simulink model "CtrlStrct_CAN_Variant"  (R2018a)
settings: Solver=VariableStepAuto  StartTime=0.0  StopTime=10.0  FixedStep=sampletime  RelTol=1e-3  EnableMultiTasking=on
PreLoadFcn:
  | CtrlStrct_SmplCAN_BusInfo
undefined symbols (not defined in the file or in its folder): canChannel
libraries: canmsglib x106, canlib x35, simulink x1
(part 2 of 8)

== system CtrlStrct_CAN_Variant/CAN_Variant/Simple_CAN_TW/HEV_Ctrl ==
  note: HEV control
  note: HEV control
  note: CAN receive and transmit
  Bus Creator1 : BusCreator  Inputs=13
  Bus Selector3 : BusSelector  OutputSignals=BatteryCtrl_PwtrCAN_Tx.BatCtrl_SOC,TransmCtrl_PwtrCAN_Tx.TmCtrl_Clutch_position,TransmCtrl_PwtrCAN_Tx.TmCtrl_Gear_position,Gateway_PwtrCAN_Tx.BrkCtrl_Vehicle_speed,Gateway_PwtrCAN_Tx.BrkCtrl_Regen_brake_torque_request,MotorCtrl_PwtrCAN_Tx.MtrCtrl_Motor_torque_actual,MotorCtrl_PwtrCAN_Tx.MtrCtrl_Motor_torque_available,MotorCtrl_PwtrCAN_Tx.MtrCtrl_Motor_regen_torque_available,EngineCtrl_PwtrCAN_Tx.EngCtrl_Engine_speed,EngineCtrl_PwtrCAN_Tx.EngCtrl_Engine_torque_actual,Gateway_PwtrCAN_Tx.VMCtrl_PropTorqStatus,Gateway_PwtrCAN_Tx.VMCtrl_PropTorqCmnd,Gateway_PwtrCAN_Tx.NAVI_Home_around_status
  Rate Transition1 : RateTransition  Deterministic=off
      settings: AttributesFormatString=<Deterministic=%<Deterministic>>
  Rate Transition2 : RateTransition  Deterministic=off
      settings: AttributesFormatString=<Deterministic=%<Deterministic>>
  Two-Way Connection : TwoWayConnection
  HevCtrl_PwtrCAN : PMIOPort  Side=Left
      settings: AttributesFormatString=<Side=%<Side>>
  tag scope: HEV_Ctrl_PwtrCAN_Rx=scoped
  wires:
  [HEV_Ctrl_PwtrCAN_Tx] -> Rate Transition2/1
  Bus Creator1/1 -> Rate Transition1/1
  Two-Way Connection/1 -> Bus Selector3/1
  Rate Transition1/1 -> [HEV_Ctrl_PwtrCAN_Rx]  "HEV_Ctrl_PwtrCAN_Rx"
  Rate Transition2/1 -> Two-Way Connection/1  "HEV_Ctrl_PwtrCAN_Tx"
  Bus Selector3/1 -> Bus Creator1/1  "<BatCtrl_SOC>"
  Bus Selector3/2 -> Bus Creator1/2  "<TmCtrl_Clutch_position>"
  Bus Selector3/3 -> Bus Creator1/3  "<TmCtrl_Gear_position>"
  Bus Selector3/4 -> Bus Creator1/4  "<BrkCtrl_Vehicle_speed>"
  Bus Selector3/5 -> Bus Creator1/5  "<BrkCtrl_Regen_brake_torque_request>"
  Bus Selector3/6 -> Bus Creator1/6  "<MtrCtrl_Motor_torque_actual>"
  Bus Selector3/7 -> Bus Creator1/7  "<MtrCtrl_Motor_torque_available>"
  Bus Selector3/8 -> Bus Creator1/8  "<MtrCtrl_Motor_regen_torque_available>"
  Bus Selector3/9 -> Bus Creator1/9  "<EngCtrl_Engine_speed>"
  Bus Selector3/10 -> Bus Creator1/10  "<EngCtrl_Engine_torque_actual>"
  Bus Selector3/11 -> Bus Creator1/11  "<VMCtrl_PropTorqStatus>"
  Bus Selector3/12 -> Bus Creator1/12  "<VMCtrl_PropTorqCmnd>"
  Bus Selector3/13 -> Bus Creator1/13  "<NAVI_Home_around_status>"
  connections:
  HevCtrl_PwtrCAN/RConn1 -- Two-Way Connection/RConn1

== system CtrlStrct_CAN_Variant/CAN_Variant/Simple_CAN_TW/HVAC_Ctrl ==
  note: HVAC control
  note: CAN receive and transmit
  note: HVAC Control
  Bus Creator : BusCreator  Inputs=3
  Bus Selector : BusSelector  OutputSignals=Gateway_VehCAN_Tx.EngCtrl_Engine_speed,Gateway_VehCAN_Tx.HEVCtrl_IdleStop_preparation_request,Gateway_VehCAN_Tx.HEVCtrl_IdleStop_status
  Rate Transition1 : RateTransition  Deterministic=off
      settings: AttributesFormatString=<Deterministic=%<Deterministic>>
  Rate Transition2 : RateTransition  Deterministic=off
      settings: AttributesFormatString=<Deterministic=%<Deterministic>>
  Two-Way Connection : TwoWayConnection
  HVAC_Ctrl_VehCAN : PMIOPort  Side=Right
      settings: AttributesFormatString=<Side=%<Side>>
  tag scope: HVAC_Ctrl_VehCAN_Rx=scoped
  wires:
  [HVAC_Ctrl_VehCAN_Tx] -> Rate Transition2/1
  Bus Creator/1 -> Rate Transition1/1
  Two-Way Connection/1 -> Bus Selector/1
  Rate Transition1/1 -> [HVAC_Ctrl_VehCAN_Rx]  "HVAC_Ctrl_VehCAN_Rx"
  Rate Transition2/1 -> Two-Way Connection/1  "HVAC_Ctrl_VehCAN_Tx"
  Bus Selector/3 -> Bus Creator/3  "<HEVCtrl_IdleStop_status>"
  Bus Selector/2 -> Bus Creator/2  "<HEVCtrl_IdleStop_preparation_request>"
  Bus Selector/1 -> Bus Creator/1  "<EngCtrl_Engine_speed>"
  connections:
  HVAC_Ctrl_VehCAN/RConn1 -- Two-Way Connection/RConn1

== system CtrlStrct_CAN_Variant/CAN_Variant/Simple_CAN_TW/InfoCAN ==
  note: Infotainment CAN
  Bus Creator : BusCreator  Inputs=3
  InfoCAN_Memory : Memory
  Two-Way Connection : TwoWayConnection
  Two-Way Connection1 : TwoWayConnection
  Two-Way Connection2 : TwoWayConnection
  NAVI_InfoCAN : PMIOPort  Side=Left
      settings: AttributesFormatString=<Side=%<Side>>
  Radar_InfoCAN : PMIOPort  Port=2  Side=Left
      settings: AttributesFormatString=<Side=%<Side>>
  Gateway_InfoCAN : PMIOPort  Port=3  Side=Right
      settings: AttributesFormatString=<Side=%<Side>>
  wires:
  Bus Creator/1 -> InfoCAN_Memory/1  "InfoCAN"
  InfoCAN_Memory/1 -> Two-Way Connection1/1, Two-Way Connection/1, Two-Way Connection2/1  "InfoCAN"
  Two-Way Connection/1 -> Bus Creator/2
  Two-Way Connection1/1 -> Bus Creator/3
  Two-Way Connection2/1 -> Bus Creator/1
  connections:
  Two-Way Connection/RConn1 -- NAVI_InfoCAN/RConn1
  Two-Way Connection1/RConn1 -- Radar_InfoCAN/RConn1
  Two-Way Connection2/RConn1 -- Gateway_InfoCAN/RConn1

== system CtrlStrct_CAN_Variant/CAN_Variant/Simple_CAN_TW/Motor_Ctrl ==
  note: Motor control
  note: Motor Control
  note: CAN receive and transmit
  Bus Creator7 : BusCreator  Inputs=3
  Bus Selector2 : BusSelector  OutputSignals=TransmCtrl_PwtrCAN_Tx.TmCtrl_Clutch_position,HEV_Ctrl_PwtrCAN_Tx.HEVCtrl_Motor_torque_request,EngineCtrl_PwtrCAN_Tx.EngCtrl_Engine_speed
  Rate Transition1 : RateTransition  Deterministic=off
      settings: AttributesFormatString=<Deterministic=%<Deterministic>>
  Rate Transition2 : RateTransition  Deterministic=off
      settings: AttributesFormatString=<Deterministic=%<Deterministic>>
  Two-Way Connection : TwoWayConnection
  MtrCtrl_PwtrCAN : PMIOPort  Side=Left
      settings: AttributesFormatString=<Side=%<Side>>
  tag scope: MotorCtrl_PwtrCAN_Rx=scoped
  wires:
  [MotorCtrl_PwtrCAN_Tx] -> Rate Transition2/1
  Rate Transition1/1 -> [MotorCtrl_PwtrCAN_Rx]  "MotorCtrl_PwtrCAN_Rx"
  Bus Selector2/3 -> Bus Creator7/3  "<EngCtrl_Engine_speed>"
  Bus Creator7/1 -> Rate Transition1/1
  Bus Selector2/1 -> Bus Creator7/1  "<TmCtrl_Clutch_position>"
  Bus Selector2/2 -> Bus Creator7/2  "<HEVCtrl_Motor_torque_request>"
  Two-Way Connection/1 -> Bus Selector2/1
  Rate Transition2/1 -> Two-Way Connection/1  "MotorCtrl_PwtrCAN_Tx"
  connections:
  MtrCtrl_PwtrCAN/RConn1 -- Two-Way Connection/RConn1

== system CtrlStrct_CAN_Variant/CAN_Variant/Simple_CAN_TW/NAVI ==
  note: Navigation
  note: Navigation
  note: CAN receive and transmit
  Bus Creator : BusCreator  Inputs=1
  Bus Selector1 : BusSelector  OutputSignals=Gateway_InfoCAN_Tx.BrkCtrl_Vehicle_speed
  Rate Transition1 : RateTransition  Deterministic=off
      settings: AttributesFormatString=<Deterministic=%<Deterministic>>
  Rate Transition2 : RateTransition  Deterministic=off
      settings: AttributesFormatString=<Deterministic=%<Deterministic>>
  Two-Way Connection : TwoWayConnection
  NAVI_InfoCAN : PMIOPort  Side=Right
      settings: AttributesFormatString=<Side=%<Side>>
  tag scope: NAVI_InfoCAN_Rx=scoped
  wires:
  [NAVI_InfoCAN_Tx] -> Rate Transition2/1
  Two-Way Connection/1 -> Bus Selector1/1
  Bus Selector1/1 -> Bus Creator/1  "<BrkCtrl_Vehicle_speed>"
  Bus Creator/1 -> Rate Transition1/1
  Rate Transition1/1 -> [NAVI_InfoCAN_Rx]  "NAVI_InfoCAN_Rx"
  Rate Transition2/1 -> Two-Way Connection/1  "NAVI_InfoCAN_Tx"
  connections:
  NAVI_InfoCAN/RConn1 -- Two-Way Connection/RConn1

== system CtrlStrct_CAN_Variant/CAN_Variant/Simple_CAN_TW/PwtrCAN ==
  note: Powertrain CAN
  Bus Creator3 : BusCreator  Inputs=6
  PwtrCAN_Memory : Memory
  Two-Way Connection{,1..5} (6 alike) : TwoWayConnection
  Gateway_PwtrCAN : PMIOPort  Side=Left
      settings: AttributesFormatString=<Side=%<Side>>
  HevCtrl_PwtrCAN : PMIOPort  Port=2  Side=Right
      settings: AttributesFormatString=<Side=%<Side>>
  EngCtrl_PwtrCAN : PMIOPort  Port=3  Side=Right
      settings: AttributesFormatString=<Side=%<Side>>
  TrsmCtrl_PwtrCAN : PMIOPort  Port=4  Side=Right
      settings: AttributesFormatString=<Side=%<Side>>
  MtrCtrl_PwtrCAN : PMIOPort  Port=5  Side=Right
      settings: AttributesFormatString=<Side=%<Side>>
  BatCtrl_PwtrCAN : PMIOPort  Port=6  Side=Right
      settings: AttributesFormatString=<Side=%<Side>>
  wires:
  Bus Creator3/1 -> PwtrCAN_Memory/1  "PwtrCAN"
  PwtrCAN_Memory/1 -> Two-Way Connection5/1, Two-Way Connection4/1, Two-Way Connection3/1, Two-Way Connection2/1, Two-Way Connection1/1, Two-Way Connection/1  "PwtrCAN"
  Two-Way Connection1/1 -> Bus Creator3/2
  Two-Way Connection/1 -> Bus Creator3/1
  Two-Way Connection2/1 -> Bus Creator3/3
  Two-Way Connection5/1 -> Bus Creator3/6
  Two-Way Connection4/1 -> Bus Creator3/5
  Two-Way Connection3/1 -> Bus Creator3/4
  connections:
  Two-Way Connection/RConn1 -- Gateway_PwtrCAN/RConn1
  HevCtrl_PwtrCAN/RConn1 -- Two-Way Connection1/RConn1
  EngCtrl_PwtrCAN/RConn1 -- Two-Way Connection2/RConn1
  Two-Way Connection3/RConn1 -- TrsmCtrl_PwtrCAN/RConn1
  MtrCtrl_PwtrCAN/RConn1 -- Two-Way Connection4/RConn1
  BatCtrl_PwtrCAN/RConn1 -- Two-Way Connection5/RConn1

== system CtrlStrct_CAN_Variant/CAN_Variant/Simple_CAN_TW/Radar ==
  note: Radar detection
  note: CAN receive and transmit
  note: Radar Detection
  Bus Creator : BusCreator  Inputs=1
  Bus Selector1 : BusSelector  OutputSignals=Gateway_InfoCAN_Tx.BrkCtrl_Vehicle_speed
  Rate Transition1 : RateTransition  Deterministic=off
      settings: AttributesFormatString=<Deterministic=%<Deterministic>>
  Rate Transition2 : RateTransition  Deterministic=off
      settings: AttributesFormatString=<Deterministic=%<Deterministic>>
  Two-Way Connection : TwoWayConnection
  Radar_InfoCAN : PMIOPort  Side=Right
      settings: AttributesFormatString=<Side=%<Side>>
  tag scope: Radar_InfoCAN_Rx=scoped
  wires:
  [Radar_InfoCAN_Tx] -> Rate Transition2/1
  Bus Selector1/1 -> Bus Creator/1  "<BrkCtrl_Vehicle_speed>"
  Bus Creator/1 -> Rate Transition1/1
  Two-Way Connection/1 -> Bus Selector1/1
  Rate Transition1/1 -> [Radar_InfoCAN_Rx]  "Radar_InfoCAN_Rx"
  Rate Transition2/1 -> Two-Way Connection/1  "Radar_InfoCAN_Tx"
  connections:
  Radar_InfoCAN/RConn1 -- Two-Way Connection/RConn1

== system CtrlStrct_CAN_Variant/CAN_Variant/Simple_CAN_TW/Steer_Ctrl ==
  note: Steering control
  note: CAN receive and transmit
  note: Steering Control
  Bus Creator : BusCreator  Inputs=1
  Bus Selector1 : BusSelector  OutputSignals=BrakeCtrl_VehCAN_Tx.BrkCtrl_Vehicle_speed
  Rate Transition1 : RateTransition  Deterministic=off
      settings: AttributesFormatString=<Deterministic=%<Deterministic>>
  Rate Transition2 : RateTransition  Deterministic=off
      settings: AttributesFormatString=<Deterministic=%<Deterministic>>
  Two-Way Connection : TwoWayConnection
  StrCtrl_VehCAN : PMIOPort  Side=Right
      settings: AttributesFormatString=<Side=%<Side>>
  tag scope: SteerCtrl_VehCAN_Rx=scoped
  wires:
  [SteerCtrl_VehCAN_Tx] -> Rate Transition2/1
  Bus Selector1/1 -> Bus Creator/1  "<BrkCtrl_Vehicle_speed>"
  Bus Creator/1 -> Rate Transition1/1
  Two-Way Connection/1 -> Bus Selector1/1
  Rate Transition1/1 -> [SteerCtrl_VehCAN_Rx]  "SteerCtrl_VehCAN_Rx"
  Rate Transition2/1 -> Two-Way Connection/1  "SteerCtrl_VehCAN_Tx"
  connections:
  StrCtrl_VehCAN/RConn1 -- Two-Way Connection/RConn1

== system CtrlStrct_CAN_Variant/CAN_Variant/Simple_CAN_TW/Transms_Ctrl ==
  note: Transmission control
  note: Transmission Control
  note: CAN receive and transmit
  Bus Creator6 : BusCreator  Inputs=2
  Bus Selector1 : BusSelector  OutputSignals=Gateway_PwtrCAN_Tx.BrkCtrl_Vehicle_speed,EngineCtrl_PwtrCAN_Tx.EngCtrl_Engine_speed
  Rate Transition1 : RateTransition  Deterministic=off
      settings: AttributesFormatString=<Deterministic=%<Deterministic>>
  Rate Transition2 : RateTransition  Deterministic=off
      settings: AttributesFormatString=<Deterministic=%<Deterministic>>
  Two-Way Connection : TwoWayConnection
  TrsmCtrl_PwtrCAN : PMIOPort  Side=Left
      settings: AttributesFormatString=<Side=%<Side>>
  tag scope: TransmCtrl_PwtrCAN_Rx=scoped
  wires:
  [TransmCtrl_PwtrCAN_Tx] -> Rate Transition2/1
  Rate Transition2/1 -> Two-Way Connection/1  "TransmCtrl_PwtrCAN_Tx"
  Bus Selector1/1 -> Bus Creator6/1  "<BrkCtrl_Vehicle_speed>"
  Bus Creator6/1 -> Rate Transition1/1
  Bus Selector1/2 -> Bus Creator6/2  "<EngCtrl_Engine_speed>"
  Two-Way Connection/1 -> Bus Selector1/1
  Rate Transition1/1 -> [TransmCtrl_PwtrCAN_Rx]  "TransmCtrl_PwtrCAN_Rx"
  connections:
  TrsmCtrl_PwtrCAN/RConn1 -- Two-Way Connection/RConn1

== system CtrlStrct_CAN_Variant/CAN_Variant/Simple_CAN_TW/VM_Ctrl ==
  note: Vehicle motion control
  note: Vehicle Motion Control
  note: CAN receive and transmit
  Bus Creator : BusCreator  Inputs=1
  Bus Selector1 : BusSelector  OutputSignals=BrakeCtrl_VehCAN_Tx.BrkCtrl_Vehicle_speed
  Rate Transition1 : RateTransition  Deterministic=off
      settings: AttributesFormatString=<Deterministic=%<Deterministic>>
  Rate Transition2 : RateTransition  Deterministic=off
      settings: AttributesFormatString=<Deterministic=%<Deterministic>>
  Two-Way Connection : TwoWayConnection
  VM_Ctrl_VehCAN : PMIOPort  Side=Right
      settings: AttributesFormatString=<Side=%<Side>>
  tag scope: VM_Ctrl_VehCAN_Rx=scoped
  wires:
  [VM_Ctrl_VehCAN_Tx] -> Rate Transition2/1
  Bus Selector1/1 -> Bus Creator/1  "<BrkCtrl_Vehicle_speed>"
  Bus Creator/1 -> Rate Transition1/1
  Two-Way Connection/1 -> Bus Selector1/1
  Rate Transition1/1 -> [VM_Ctrl_VehCAN_Rx]  "VM_Ctrl_VehCAN_Rx"
  Rate Transition2/1 -> Two-Way Connection/1  "VM_Ctrl_VehCAN_Tx"
  connections:
  VM_Ctrl_VehCAN/RConn1 -- Two-Way Connection/RConn1

== system CtrlStrct_CAN_Variant/CAN_Variant/Simple_CAN_TW/VehCAN ==
  note: Vehicle CAN
  Bus Creator1 : BusCreator  Inputs=6
  Two-Way Connection{,1..5} (6 alike) : TwoWayConnection
  VehCAN_Memory : Memory
  Gateway_VehCAN : PMIOPort  Side=Right
      settings: AttributesFormatString=<Side=%<Side>>
  VM_Ctrl_VehCAN : PMIOPort  Port=2  Side=Left
      settings: AttributesFormatString=<Side=%<Side>>
  BrkCtrl_VehCAN : PMIOPort  Port=3  Side=Left
      settings: AttributesFormatString=<Side=%<Side>>
  StrCtrl_VehCAN : PMIOPort  Port=4  Side=Left
      settings: AttributesFormatString=<Side=%<Side>>
  HVAC_Ctrl_VehCAN : PMIOPort  Port=5  Side=Left
      settings: AttributesFormatString=<Side=%<Side>>
  BdyCtrl_VehCAN : PMIOPort  Port=6  Side=Left
      settings: AttributesFormatString=<Side=%<Side>>
  wires:
  Bus Creator1/1 -> VehCAN_Memory/1  "VehCAN"
  Two-Way Connection3/1 -> Bus Creator1/4
  Two-Way Connection1/1 -> Bus Creator1/2
  Two-Way Connection5/1 -> Bus Creator1/6
  VehCAN_Memory/1 -> Two-Way Connection/1, Two-Way Connection3/1, Two-Way Connection2/1, Two-Way Connection1/1, Two-Way Connection4/1, Two-Way Connection5/1  "VehCAN"
  Two-Way Connection2/1 -> Bus Creator1/3
  Two-Way Connection/1 -> Bus Creator1/1
  Two-Way Connection4/1 -> Bus Creator1/5
  connections:
  Gateway_VehCAN/RConn1 -- Two-Way Connection/RConn1
  Two-Way Connection1/RConn1 -- VM_Ctrl_VehCAN/RConn1
  Two-Way Connection2/RConn1 -- BrkCtrl_VehCAN/RConn1
  Two-Way Connection3/RConn1 -- StrCtrl_VehCAN/RConn1
  Two-Way Connection4/RConn1 -- HVAC_Ctrl_VehCAN/RConn1
  BdyCtrl_VehCAN/RConn1 -- Two-Way Connection5/RConn1

== system CtrlStrct_CAN_Variant/CAN_Variant/VNT_Level1_CAN_TW/Battery_Ctrl ==
  note: Battery control
  note: CAN receive and transmit
  note: Battery Control
  BatteryCtrl_PwtrCAN Tx : Subsystem
  BatteryCtrl_PwtrCAN_Rx : Subsystem
  Two-Way Connection : TwoWayConnection
  BatCtrl_PwtrCAN : PMIOPort  Side=Left
      settings: AttributesFormatString=<Side=%<Side>>
  tag scope: BatteryCtrl_PwtrCAN_Rx=scoped
  wires:
  [BatteryCtrl_PwtrCAN_Tx] -> BatteryCtrl_PwtrCAN Tx/1(BatteryCtrl_PwtrCAN_Tx_Apli)
  BatteryCtrl_PwtrCAN_Rx/1(BatteryCtrl_PwtrCAN_Rx) -> [BatteryCtrl_PwtrCAN_Rx]
  Two-Way Connection/1 -> BatteryCtrl_PwtrCAN_Rx/1(PwtrCAN)
  BatteryCtrl_PwtrCAN Tx/1(BatteryCtrl_PwtrCAN_Tx) -> Two-Way Connection/1
  connections:
  BatCtrl_PwtrCAN/RConn1 -- Two-Way Connection/RConn1

== system CtrlStrct_CAN_Variant/CAN_Variant/VNT_Level1_CAN_TW/Body_Ctrl ==
  note: Body control
  note: Body Control
  note: CAN receive and transmit
  BodyCtrl_VehCAN Tx : Subsystem
  BodyCtrl_VehCAN_Rx : Subsystem
  Two-Way Connection : TwoWayConnection
  BdyCtrl_VehCAN : PMIOPort  Side=Right
      settings: AttributesFormatString=<Side=%<Side>>
  tag scope: BodyCtrl_VehCAN_Rx=scoped
  wires:
  [BodyCtrl_VehCAN_Tx] -> BodyCtrl_VehCAN Tx/1(BodyCtrl_VehCAN_Tx_Apli)
  BodyCtrl_VehCAN_Rx/1(BodyCtrl_VehCAN_Rx) -> [BodyCtrl_VehCAN_Rx]
  Two-Way Connection/1 -> BodyCtrl_VehCAN_Rx/1(VehCAN)
  BodyCtrl_VehCAN Tx/1(BodyCtrl_VehCAN_Tx) -> Two-Way Connection/1
  connections:
  BdyCtrl_VehCAN/RConn1 -- Two-Way Connection/RConn1

== system CtrlStrct_CAN_Variant/CAN_Variant/VNT_Level1_CAN_TW/Brake_Ctrl ==
  note: Brake control
  note: Brake Control
  note: CAN receive and transmit
  BrakeCtrl_VehCAN Tx : Subsystem
  BrakeCtrl_VehCAN_Rx : Subsystem
  Two-Way Connection : TwoWayConnection
  BrkCtrl_VehCAN : PMIOPort  Side=Right
      settings: AttributesFormatString=<Side=%<Side>>
  tag scope: BrakeCtrl_VehCAN_Rx=scoped
  wires:
  [BrakeCtrl_VehCAN_Tx] -> BrakeCtrl_VehCAN Tx/1(BrakeCtrl_VehCAN_Tx_Apli)
  BrakeCtrl_VehCAN_Rx/1(BrakeCtrl_VehCAN_Rx) -> [BrakeCtrl_VehCAN_Rx]
  Two-Way Connection/1 -> BrakeCtrl_VehCAN_Rx/1(VehCAN)
  BrakeCtrl_VehCAN Tx/1(BrakeCtrl_VehCAN_Tx) -> Two-Way Connection/1
  connections:
  BrkCtrl_VehCAN/RConn1 -- Two-Way Connection/RConn1

== system CtrlStrct_CAN_Variant/CAN_Variant/VNT_Level1_CAN_TW/Engine_Ctrl ==
  note: Engine control
  note: Engine Control
  note: CAN receive and transmit
  EngineCtrl_PwtrCAN Tx : Subsystem
  EngineCtrl_PwtrCAN_Rx : Subsystem
  Two-Way Connection : TwoWayConnection
  EngCtrl_PwtrCAN : PMIOPort  Side=Left
      settings: AttributesFormatString=<Side=%<Side>>
  tag scope: EngineCtrl_PwtrCAN_Rx=scoped
  wires:
  [EngineCtrl_PwtrCAN_Tx] -> EngineCtrl_PwtrCAN Tx/1(EngineCtrl_PwtrCAN_Tx_Apli)
  EngineCtrl_PwtrCAN_Rx/1(EngineCtrl_PwtrCAN_Rx) -> [EngineCtrl_PwtrCAN_Rx]
  Two-Way Connection/1 -> EngineCtrl_PwtrCAN_Rx/1(PwtrCAN)
  EngineCtrl_PwtrCAN Tx/1(EngineCtrl_PwtrCAN_Tx) -> Two-Way Connection/1
  connections:
  EngCtrl_PwtrCAN/RConn1 -- Two-Way Connection/RConn1

== system CtrlStrct_CAN_Variant/CAN_Variant/VNT_Level1_CAN_TW/Gateway ==
  note: Gateway
  Gateway InfoCAN : Subsystem
  Gateway PwtrCAN : Subsystem
  Gateway VehCAN : Subsystem
  Info Hub : Subsystem
  Two-Way Connection : TwoWayConnection
  Two-Way Connection1 : TwoWayConnection
  Two-Way Connection2 : TwoWayConnection
  Gateway_InfoCAN : PMIOPort  Side=Left
      settings: AttributesFormatString=<Side=%<Side>>
  Gateway_VehCAN : PMIOPort  Port=2  Side=Left
      settings: AttributesFormatString=<Side=%<Side>>
  Gateway_PwtrCAN : PMIOPort  Port=3  Side=Right
      settings: AttributesFormatString=<Side=%<Side>>
  wires:
  Two-Way Connection1/1 -> Gateway PwtrCAN/2(VehCAN), Gateway InfoCAN/1(VehCAN), Info Hub/2(VehCAN)
  Two-Way Connection2/1 -> Gateway VehCAN/2(PwtrCAN), Info Hub/3(PwtrCAN)
  Two-Way Connection/1 -> Gateway VehCAN/1(InfoCAN), Gateway PwtrCAN/1(InfoCAN), Info Hub/1(InfoCAN)
  Gateway InfoCAN/1(Gateway_InfoCAN) -> Two-Way Connection/1
  Gateway VehCAN/1(Gateway_VehCAN_Tx) -> Two-Way Connection1/1
  Gateway PwtrCAN/1(Gateway_PwtrCAN_Tx) -> Two-Way Connection2/1
  connections:
  Gateway_InfoCAN/RConn1 -- Two-Way Connection/RConn1
  Two-Way Connection1/RConn1 -- Gateway_VehCAN/RConn1
  Gateway_PwtrCAN/RConn1 -- Two-Way Connection2/RConn1

== system CtrlStrct_CAN_Variant/CAN_Variant/VNT_Level1_CAN_TW/HEV_Ctrl ==
  note: HEV control
  note: HEV control
  note: CAN receive and transmit
  HEV_Ctrl_PwtrCAN Tx : Subsystem
  HEV_Ctrl_PwtrCAN_Rx : Subsystem
  Two-Way Connection : TwoWayConnection
  HevCtrl_PwtrCAN : PMIOPort  Side=Left
      settings: AttributesFormatString=<Side=%<Side>>
  tag scope: HEV_Ctrl_PwtrCAN_Rx=scoped
  wires:
  [HEV_Ctrl_PwtrCAN_Tx] -> HEV_Ctrl_PwtrCAN Tx/1(HEV_Ctrl_PwtrCAN_Tx_Apli)
  Two-Way Connection/1 -> HEV_Ctrl_PwtrCAN_Rx/1(PwtrCAN)
  HEV_Ctrl_PwtrCAN_Rx/1(HEV_Ctrl_PwtrCAN_Rx) -> [HEV_Ctrl_PwtrCAN_Rx]
  HEV_Ctrl_PwtrCAN Tx/1(HEV_Ctrl_PwtrCAN_Tx) -> Two-Way Connection/1
  connections:
  HevCtrl_PwtrCAN/RConn1 -- Two-Way Connection/RConn1

== system CtrlStrct_CAN_Variant/CAN_Variant/VNT_Level1_CAN_TW/HVAC_Ctrl ==
  note: HVAC control
  note: CAN receive and transmit
  note: HVAC Control
  HVAC_Ctrl_VehCAN Tx : Subsystem
  HVAC_Ctrl_VehCAN_Rx : Subsystem
  Two-Way Connection : TwoWayConnection
  HVAC_Ctrl_VehCAN : PMIOPort  Side=Right
      settings: AttributesFormatString=<Side=%<Side>>
  tag scope: HVAC_Ctrl_VehCAN_Rx=scoped
  wires:
  [HVAC_Ctrl_VehCAN_Tx] -> HVAC_Ctrl_VehCAN Tx/1(HVAC_Ctrl_VehCAN_Tx_Apli)
  Two-Way Connection/1 -> HVAC_Ctrl_VehCAN_Rx/1(VehCAN)
  HVAC_Ctrl_VehCAN_Rx/1(HVAC_Ctrl_VehCAN_Rx) -> [HVAC_Ctrl_VehCAN_Rx]
  HVAC_Ctrl_VehCAN Tx/1(HVAC_Ctrl_VehCAN_Tx) -> Two-Way Connection/1
  connections:
  HVAC_Ctrl_VehCAN/RConn1 -- Two-Way Connection/RConn1

== system CtrlStrct_CAN_Variant/CAN_Variant/VNT_Level1_CAN_TW/InfoCAN ==
  note: Infotainment CAN
  Bus Creator : BusCreator  Inputs=3
  Bus Selector : BusSelector  OutputSignals=NAVI_InfoCAN_Tx_0CFFB01C
  Bus Selector1 : BusSelector  OutputSignals=Gateway_InfoCAN_Tx_0CFFC485
  Bus Selector2 : BusSelector  OutputSignals=Radar_InfoCAN_Tx_0CFF0080
  CAN_Memory : Memory
  Two-Way Connection : TwoWayConnection
  Two-Way Connection1 : TwoWayConnection
  Two-Way Connection2 : TwoWayConnection
  NAVI_InfoCAN : PMIOPort  Side=Left
      settings: AttributesFormatString=<Side=%<Side>>
  Radar_InfoCAN : PMIOPort  Port=2  Side=Left
      settings: AttributesFormatString=<Side=%<Side>>
  Gateway_InfoCAN : PMIOPort  Port=3  Side=Right
      settings: AttributesFormatString=<Side=%<Side>>
  wires:
  Bus Creator/1 -> CAN_Memory/1  "InfoCAN"
  CAN_Memory/1 -> Two-Way Connection2/1, Two-Way Connection1/1, Two-Way Connection/1  "InfoCAN"
  Two-Way Connection/1 -> Bus Selector/1
  Two-Way Connection1/1 -> Bus Selector2/1
  Two-Way Connection2/1 -> Bus Selector1/1
  Bus Selector1/1 -> Bus Creator/1  "<Gateway_InfoCAN_Tx_0CFFC485>"
  Bus Selector/1 -> Bus Creator/2  "<NAVI_InfoCAN_Tx_0CFFB01C>"
  Bus Selector2/1 -> Bus Creator/3  "<Radar_InfoCAN_Tx_0CFF0080>"
  connections:
  Two-Way Connection/RConn1 -- NAVI_InfoCAN/RConn1
  Two-Way Connection1/RConn1 -- Radar_InfoCAN/RConn1
  Two-Way Connection2/RConn1 -- Gateway_InfoCAN/RConn1

== system CtrlStrct_CAN_Variant/CAN_Variant/VNT_Level1_CAN_TW/Motor_Ctrl ==
  note: Motor control
  note: Motor Control
  note: CAN receive and transmit
  MotorCtrl_PwtrCAN Tx : Subsystem
  MotorCtrl_PwtrCAN_Rx : Subsystem
  Two-Way Connection : TwoWayConnection
  MtrCtrl_PwtrCAN : PMIOPort  Side=Left
      settings: AttributesFormatString=<Side=%<Side>>
  tag scope: MotorCtrl_PwtrCAN_Rx=scoped
  wires:
  [MotorCtrl_PwtrCAN_Tx] -> MotorCtrl_PwtrCAN Tx/1(IMotorCtrl_PwtrCAN_Tx_Apli)
  Two-Way Connection/1 -> MotorCtrl_PwtrCAN_Rx/1(PwtrCAN)
  MotorCtrl_PwtrCAN_Rx/1(MotorCtrl_PwtrCAN_Rx) -> [MotorCtrl_PwtrCAN_Rx]
  MotorCtrl_PwtrCAN Tx/1(MotorCtrl_PwtrCAN_Tx_0CFF5083) -> Two-Way Connection/1
  connections:
  MtrCtrl_PwtrCAN/RConn1 -- Two-Way Connection/RConn1

== system CtrlStrct_CAN_Variant/CAN_Variant/VNT_Level1_CAN_TW/NAVI ==
  note: Navigation
  note: Navigation
  note: CAN receive and transmit
  NAVI_InfoCAN_Rx : Subsystem
  NAVI_InfoCAN_Tx : Subsystem
  Two-Way Connection : TwoWayConnection
  NAVI_InfoCAN : PMIOPort  Side=Right
      settings: AttributesFormatString=<Side=%<Side>>
  tag scope: NAVI_InfoCAN_Rx=scoped
  wires:
  Two-Way Connection/1 -> NAVI_InfoCAN_Rx/1(InfoCAN)
  NAVI_InfoCAN_Rx/1(NAVI_InfoCAN_Rx) -> [NAVI_InfoCAN_Rx]
  [NAVI_InfoCAN_Tx] -> NAVI_InfoCAN_Tx/1(NAVI_InfoCAN_Tx_Apli)
  NAVI_InfoCAN_Tx/1(NAVI_InfoCAN_Tx) -> Two-Way Connection/1
  connections:
  NAVI_InfoCAN/RConn1 -- Two-Way Connection/RConn1

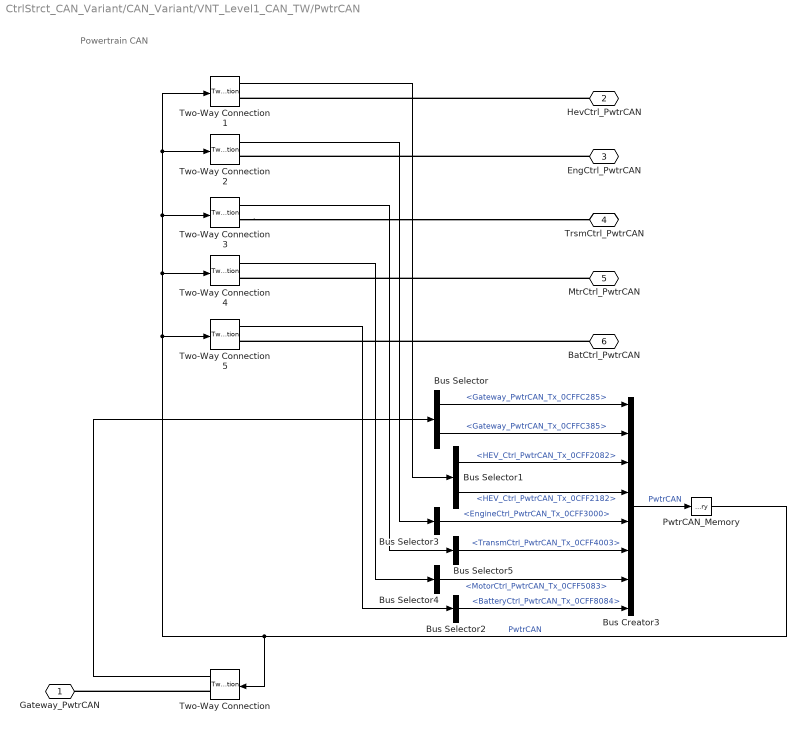
== system CtrlStrct_CAN_Variant/CAN_Variant/VNT_Level1_CAN_TW/PwtrCAN ==
  note: Powertrain CAN
  Bus Creator3 : BusCreator  Inputs=8
  Bus Selector : BusSelector  OutputSignals=Gateway_PwtrCAN_Tx_0CFFC285,Gateway_PwtrCAN_Tx_0CFFC385
  Bus Selector1 : BusSelector  OutputSignals=HEV_Ctrl_PwtrCAN_Tx_0CFF2082,HEV_Ctrl_PwtrCAN_Tx_0CFF2182
  Bus Selector2 : BusSelector  OutputSignals=BatteryCtrl_PwtrCAN_Tx_0CFF8084
  Bus Selector3 : BusSelector  OutputSignals=EngineCtrl_PwtrCAN_Tx_0CFF3000
  Bus Selector4 : BusSelector  OutputSignals=MotorCtrl_PwtrCAN_Tx_0CFF5083
  Bus Selector5 : BusSelector  OutputSignals=TransmCtrl_PwtrCAN_Tx_0CFF4003
  PwtrCAN_Memory : Memory
  Two-Way Connection{,1..5} (6 alike) : TwoWayConnection
  Gateway_PwtrCAN : PMIOPort  Side=Left
      settings: AttributesFormatString=<Side=%<Side>>
  HevCtrl_PwtrCAN : PMIOPort  Port=2  Side=Right
      settings: AttributesFormatString=<Side=%<Side>>
  EngCtrl_PwtrCAN : PMIOPort  Port=3  Side=Right
      settings: AttributesFormatString=<Side=%<Side>>
  TrsmCtrl_PwtrCAN : PMIOPort  Port=4  Side=Right
      settings: AttributesFormatString=<Side=%<Side>>
  MtrCtrl_PwtrCAN : PMIOPort  Port=5  Side=Right
      settings: AttributesFormatString=<Side=%<Side>>
  BatCtrl_PwtrCAN : PMIOPort  Port=6  Side=Right
      settings: AttributesFormatString=<Side=%<Side>>
  wires:
  Bus Creator3/1 -> PwtrCAN_Memory/1  "PwtrCAN"
  PwtrCAN_Memory/1 -> Two-Way Connection5/1, Two-Way Connection4/1, Two-Way Connection3/1, Two-Way Connection2/1, Two-Way Connection1/1, Two-Way Connection/1  "PwtrCAN"
  Two-Way Connection1/1 -> Bus Selector1/1
  Two-Way Connection/1 -> Bus Selector/1
  Two-Way Connection2/1 -> Bus Selector3/1
  Two-Way Connection5/1 -> Bus Selector2/1
  Two-Way Connection4/1 -> Bus Selector4/1
  Two-Way Connection3/1 -> Bus Selector5/1
  Bus Selector/1 -> Bus Creator3/1  "<Gateway_PwtrCAN_Tx_0CFFC285>"
  Bus Selector/2 -> Bus Creator3/2  "<Gateway_PwtrCAN_Tx_0CFFC385>"
  Bus Selector1/1 -> Bus Creator3/3  "<HEV_Ctrl_PwtrCAN_Tx_0CFF2082>"
  Bus Selector1/2 -> Bus Creator3/4  "<HEV_Ctrl_PwtrCAN_Tx_0CFF2182>"
  Bus Selector3/1 -> Bus Creator3/5  "<EngineCtrl_PwtrCAN_Tx_0CFF3000>"
  Bus Selector5/1 -> Bus Creator3/6  "<TransmCtrl_PwtrCAN_Tx_0CFF4003>"
  Bus Selector4/1 -> Bus Creator3/7  "<MotorCtrl_PwtrCAN_Tx_0CFF5083>"
  Bus Selector2/1 -> Bus Creator3/8  "<BatteryCtrl_PwtrCAN_Tx_0CFF8084>"
  connections:
  Two-Way Connection/RConn1 -- Gateway_PwtrCAN/RConn1
  HevCtrl_PwtrCAN/RConn1 -- Two-Way Connection1/RConn1
  EngCtrl_PwtrCAN/RConn1 -- Two-Way Connection2/RConn1
  Two-Way Connection3/RConn1 -- TrsmCtrl_PwtrCAN/RConn1
  MtrCtrl_PwtrCAN/RConn1 -- Two-Way Connection4/RConn1
  BatCtrl_PwtrCAN/RConn1 -- Two-Way Connection5/RConn1

== system CtrlStrct_CAN_Variant/CAN_Variant/VNT_Level1_CAN_TW/Radar ==
  note: Radar detection
  note: CAN receive and transmit
  note: Radar Detection
  Radar_InfoCAN_Rx : Subsystem
  Radar_InfoCAN_Tx : Subsystem
  Two-Way Connection : TwoWayConnection
  Radar_InfoCAN : PMIOPort  Side=Right
      settings: AttributesFormatString=<Side=%<Side>>
  tag scope: Radar_InfoCAN_Rx=scoped
  wires:
  Two-Way Connection/1 -> Radar_InfoCAN_Rx/1(InfoCAN)
  Radar_InfoCAN_Rx/1(Radar_InfoCAN_Rx) -> [Radar_InfoCAN_Rx]
  [Radar_InfoCAN_Tx] -> Radar_InfoCAN_Tx/1(Radar_InfoCAN_Tx_Apli)
  Radar_InfoCAN_Tx/1(Radar_InfoCAN_Tx) -> Two-Way Connection/1
  connections:
  Radar_InfoCAN/RConn1 -- Two-Way Connection/RConn1

== system CtrlStrct_CAN_Variant/CAN_Variant/VNT_Level1_CAN_TW/Steer_Ctrl ==
  note: Steering control
  note: CAN receive and transmit
  note: Steering Control
  SteerCtrl_VehCAN Tx : Subsystem
  SteerCtrl_VehCAN_Rx : Subsystem
  Two-Way Connection : TwoWayConnection
  StrCtrl_VehCAN : PMIOPort  Side=Right
      settings: AttributesFormatString=<Side=%<Side>>
  tag scope: SteerCtrl_VehCAN_Rx=scoped
  wires:
  [SteerCtrl_VehCAN_Tx] -> SteerCtrl_VehCAN Tx/1(SteerCtrl_VehCAN_Tx_Apli)
  Two-Way Connection/1 -> SteerCtrl_VehCAN_Rx/1(VehCAN)
  SteerCtrl_VehCAN_Rx/1(SteerCtrl_VehCAN_Rx) -> [SteerCtrl_VehCAN_Rx]
  SteerCtrl_VehCAN Tx/1(SteerCtrl_VehCAN_Tx) -> Two-Way Connection/1
  connections:
  StrCtrl_VehCAN/RConn1 -- Two-Way Connection/RConn1

== system CtrlStrct_CAN_Variant/CAN_Variant/VNT_Level1_CAN_TW/Transms_Ctrl ==
  note: Transmission control
  note: Transmission Control
  note: CAN receive and transmit
  TransmCtrl_PwtrCAN Tx : Subsystem
  TransmCtrl_PwtrCAN_Rx : Subsystem
  Two-Way Connection : TwoWayConnection
  TrsmCtrl_PwtrCAN : PMIOPort  Side=Left
      settings: AttributesFormatString=<Side=%<Side>>
  tag scope: TransmCtrl_PwtrCAN_Rx=scoped
  wires:
  [TransmCtrl_PwtrCAN_Tx] -> TransmCtrl_PwtrCAN Tx/1(TransmCtrl_PwtrCAN_Tx_Apli)
  Two-Way Connection/1 -> TransmCtrl_PwtrCAN_Rx/1(PwtrCAN)
  TransmCtrl_PwtrCAN_Rx/1(TransmCtrl_PwtrCAN_Rx) -> [TransmCtrl_PwtrCAN_Rx]
  TransmCtrl_PwtrCAN Tx/1(TransmCtrl_PwtrCAN_Tx) -> Two-Way Connection/1
  connections:
  TrsmCtrl_PwtrCAN/RConn1 -- Two-Way Connection/RConn1

== system CtrlStrct_CAN_Variant/CAN_Variant/VNT_Level1_CAN_TW/VM_Ctrl ==
  note: Vehicle motion control
  note: Vehicle Motion Control
  note: CAN receive and transmit
  Two-Way Connection : TwoWayConnection
  VM_Ctrl_VehCAN Tx : Subsystem
  VM_Ctrl_VehCAN_Rx : Subsystem
  VM_Ctrl_VehCAN : PMIOPort  Side=Right
      settings: AttributesFormatString=<Side=%<Side>>
  tag scope: VM_Ctrl_VehCAN_Rx=scoped
  wires:
  [VM_Ctrl_VehCAN_Tx] -> VM_Ctrl_VehCAN Tx/1(VM_Ctrl_VehCAN_Tx_Apli)
  Two-Way Connection/1 -> VM_Ctrl_VehCAN_Rx/1(VehCAN)
  VM_Ctrl_VehCAN_Rx/1(VM_Ctrl_VehCAN_Rx) -> [VM_Ctrl_VehCAN_Rx]
  VM_Ctrl_VehCAN Tx/1(VM_Ctrl_VehCAN_Tx) -> Two-Way Connection/1
  connections:
  VM_Ctrl_VehCAN/RConn1 -- Two-Way Connection/RConn1

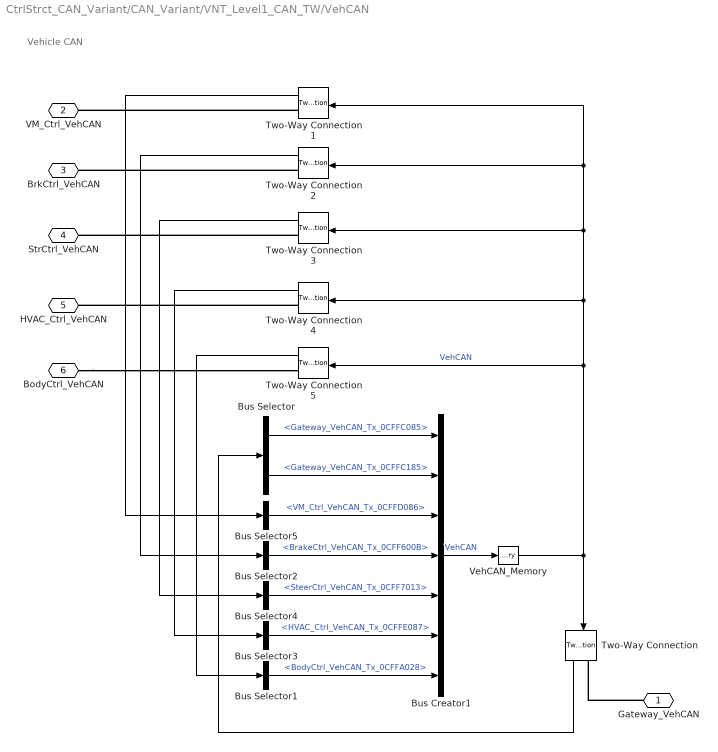
== system CtrlStrct_CAN_Variant/CAN_Variant/VNT_Level1_CAN_TW/VehCAN ==
  note: Vehicle CAN
  Bus Creator1 : BusCreator  Inputs=7
  Bus Selector : BusSelector  OutputSignals=Gateway_VehCAN_Tx_0CFFC085,Gateway_VehCAN_Tx_0CFFC185
  Bus Selector1 : BusSelector  OutputSignals=BodyCtrl_VehCAN_Tx_0CFFA028
  Bus Selector2 : BusSelector  OutputSignals=BrakeCtrl_VehCAN_Tx_0CFF600B
  Bus Selector3 : BusSelector  OutputSignals=HVAC_Ctrl_VehCAN_Tx_0CFFE087
  Bus Selector4 : BusSelector  OutputSignals=SteerCtrl_VehCAN_Tx_0CFF7013
  Bus Selector5 : BusSelector  OutputSignals=VM_Ctrl_VehCAN_Tx_0CFFD086
  Two-Way Connection{,1..5} (6 alike) : TwoWayConnection
  VehCAN_Memory : Memory
  Gateway_VehCAN : PMIOPort  Side=Right
      settings: AttributesFormatString=<Side=%<Side>>
  VM_Ctrl_VehCAN : PMIOPort  Port=2  Side=Left
      settings: AttributesFormatString=<Side=%<Side>>
  BrkCtrl_VehCAN : PMIOPort  Port=3  Side=Left
      settings: AttributesFormatString=<Side=%<Side>>
  StrCtrl_VehCAN : PMIOPort  Port=4  Side=Left
      settings: AttributesFormatString=<Side=%<Side>>
  HVAC_Ctrl_VehCAN : PMIOPort  Port=5  Side=Left
      settings: AttributesFormatString=<Side=%<Side>>
  BodyCtrl_VehCAN : PMIOPort  Port=6  Side=Left
      settings: AttributesFormatString=<Side=%<Side>>
  wires:
  Bus Creator1/1 -> VehCAN_Memory/1  "VehCAN"
  Two-Way Connection3/1 -> Bus Selector4/1
  Two-Way Connection1/1 -> Bus Selector5/1
  Two-Way Connection5/1 -> Bus Selector1/1
  VehCAN_Memory/1 -> Two-Way Connection4/1, Two-Way Connection3/1, Two-Way Connection2/1, Two-Way Connection1/1, Two-Way Connection5/1, Two-Way Connection/1  "VehCAN"
  Two-Way Connection2/1 -> Bus Selector2/1
  Two-Way Connection/1 -> Bus Selector/1
  Two-Way Connection4/1 -> Bus Selector3/1
  Bus Selector/1 -> Bus Creator1/1  "<Gateway_VehCAN_Tx_0CFFC085>"
  Bus Selector/2 -> Bus Creator1/2  "<Gateway_VehCAN_Tx_0CFFC185>"
  Bus Selector5/1 -> Bus Creator1/3  "<VM_Ctrl_VehCAN_Tx_0CFFD086>"
  Bus Selector2/1 -> Bus Creator1/4  "<BrakeCtrl_VehCAN_Tx_0CFF600B>"
  Bus Selector4/1 -> Bus Creator1/5  "<SteerCtrl_VehCAN_Tx_0CFF7013>"
  Bus Selector3/1 -> Bus Creator1/6  "<HVAC_Ctrl_VehCAN_Tx_0CFFE087>"
  Bus Selector1/1 -> Bus Creator1/7  "<BodyCtrl_VehCAN_Tx_0CFFA028>"
  connections:
  Gateway_VehCAN/RConn1 -- Two-Way Connection/RConn1
  Two-Way Connection1/RConn1 -- VM_Ctrl_VehCAN/RConn1
  Two-Way Connection2/RConn1 -- BrkCtrl_VehCAN/RConn1
  Two-Way Connection3/RConn1 -- StrCtrl_VehCAN/RConn1
  Two-Way Connection4/RConn1 -- HVAC_Ctrl_VehCAN/RConn1
  BodyCtrl_VehCAN/RConn1 -- Two-Way Connection5/RConn1

== system CtrlStrct_CAN_Variant/CAN_Variant/VNT_Level_2_CAN/Battery_Ctrl ==
  note: Battery control
  note: CAN receive and transmit
  note: Battery Control
  BatteryCtrl_PwtrCAN Tx : Subsystem
  BatteryCtrl_PwtrCAN_Rx : Subsystem
  Two-Way Connection : TwoWayConnection
  BatCtrl_PwtrCAN : PMIOPort  Side=Left
      settings: AttributesFormatString=<Side=%<Side>>
  tag scope: BatteryCtrl_PwtrCAN_Rx=scoped
  wires:
  [BatteryCtrl_PwtrCAN_Tx] -> BatteryCtrl_PwtrCAN Tx/1(BatteryCtrl_PwtrCAN_Tx_Apli)
  BatteryCtrl_PwtrCAN Tx/1(BatteryCtrl_PwtrCAN_Tx) -> Two-Way Connection/1
  Two-Way Connection/1 -> BatteryCtrl_PwtrCAN_Rx/1(PwtrCAN)
  BatteryCtrl_PwtrCAN_Rx/1(BatteryCtrl_PwtrCAN_Rx) -> [BatteryCtrl_PwtrCAN_Rx]
  connections:
  BatCtrl_PwtrCAN/RConn1 -- Two-Way Connection/RConn1

== system CtrlStrct_CAN_Variant/CAN_Variant/VNT_Level_2_CAN/Body_Ctrl ==
  note: Body Control
  note: CAN receive and transmit
  note: Body control
  BodyCtrl_VehCAN Tx : Subsystem
  BodyCtrl_VehCAN_Rx : Subsystem
  Two-Way Connection : TwoWayConnection
  BdyCtrl_VehCAN : PMIOPort  Side=Right
      settings: AttributesFormatString=<Side=%<Side>>
  tag scope: BodyCtrl_VehCAN_Rx=scoped
  wires:
  [BodyCtrl_VehCAN_Tx] -> BodyCtrl_VehCAN Tx/1(BodyCtrl_VehCAN_Tx_Apli)
  BodyCtrl_VehCAN Tx/1(BodyCtrl_VehCAN_Tx) -> Two-Way Connection/1
  Two-Way Connection/1 -> BodyCtrl_VehCAN_Rx/1(VehCAN)
  BodyCtrl_VehCAN_Rx/1(BodyCtrl_VehCAN_Rx) -> [BodyCtrl_VehCAN_Rx]
  connections:
  BdyCtrl_VehCAN/RConn1 -- Two-Way Connection/RConn1

== system CtrlStrct_CAN_Variant/CAN_Variant/VNT_Level_2_CAN/Brake_Ctrl ==
  note: Brake Control
  note: CAN receive and transmit
  note: Brake control
  BrakeCtrl_VehCAN Tx : Subsystem
  BrakeCtrl_VehCAN_Rx : Subsystem
  Two-Way Connection : TwoWayConnection
  BrkCtrl_VehCAN : PMIOPort  Side=Right
      settings: AttributesFormatString=<Side=%<Side>>
  tag scope: BrakeCtrl_VehCAN_Rx=scoped
  wires:
  [BrakeCtrl_VehCAN_Tx] -> BrakeCtrl_VehCAN Tx/1(BrakeCtrl_VehCAN_Tx_Apli)
  BrakeCtrl_VehCAN Tx/1(BrakeCtrl_VehCAN_Tx) -> Two-Way Connection/1
  Two-Way Connection/1 -> BrakeCtrl_VehCAN_Rx/1(VehCAN)
  BrakeCtrl_VehCAN_Rx/1(BrakeCtrl_VehCAN_Rx) -> [BrakeCtrl_VehCAN_Rx]
  connections:
  BrkCtrl_VehCAN/RConn1 -- Two-Way Connection/RConn1

== system CtrlStrct_CAN_Variant/CAN_Variant/VNT_Level_2_CAN/Engine_Ctrl ==
  note: Engine control
  note: Engine Control
  note: CAN receive and transmit
  EngineCtrl_PwtrCAN Tx : Subsystem
  EngineCtrl_PwtrCAN_Rx : Subsystem
  Two-Way Connection : TwoWayConnection
  EngCtrl_PwtrCAN : PMIOPort  Side=Left
      settings: AttributesFormatString=<Side=%<Side>>
  tag scope: EngineCtrl_PwtrCAN_Rx=scoped
  wires:
  [EngineCtrl_PwtrCAN_Tx] -> EngineCtrl_PwtrCAN Tx/1(EngineCtrl_PwtrCAN_Tx_Apli)
  EngineCtrl_PwtrCAN Tx/1(EngineCtrl_PwtrCAN_Tx) -> Two-Way Connection/1
  Two-Way Connection/1 -> EngineCtrl_PwtrCAN_Rx/1(PwtrCAN)
  EngineCtrl_PwtrCAN_Rx/1(EngineCtrl_PwtrCAN_Rx) -> [EngineCtrl_PwtrCAN_Rx]
  connections:
  EngCtrl_PwtrCAN/RConn1 -- Two-Way Connection/RConn1

== system CtrlStrct_CAN_Variant/CAN_Variant/VNT_Level_2_CAN/Gateway ==
  note: Gateway
  Gateway InfoCAN : Subsystem
  Gateway PwtrCAN : Subsystem
  Gateway VehCAN : Subsystem
  Info Hub : Subsystem
  Two-Way Connection : TwoWayConnection
  Two-Way Connection1 : TwoWayConnection
  Two-Way Connection2 : TwoWayConnection
  Gateway_InfoCAN : PMIOPort  Side=Left
      settings: AttributesFormatString=<Side=%<Side>>
  Gateway_VehCAN : PMIOPort  Port=2  Side=Left
      settings: AttributesFormatString=<Side=%<Side>>
  Gateway_PwtrCAN : PMIOPort  Port=3  Side=Right
      settings: AttributesFormatString=<Side=%<Side>>
  wires:
  Two-Way Connection/1 -> Gateway PwtrCAN/1(InfoCAN), Info Hub/1(InfoCAN), Gateway VehCAN/1(InfoCAN)
  Two-Way Connection2/1 -> Gateway VehCAN/2(PwtrCAN), Info Hub/3(PwtrCAN)
  Gateway InfoCAN/1(Gateway_InfoCAN) -> Two-Way Connection/1
  Gateway VehCAN/1(Gateway_VehCAN_Tx) -> Two-Way Connection1/1
  Gateway PwtrCAN/1(Gateway_PwtrCAN_Tx) -> Two-Way Connection2/1
  Two-Way Connection1/1 -> Gateway InfoCAN/1(VehCAN), Gateway PwtrCAN/2(VehCAN), Info Hub/2(VehCAN)
  Gateway PwtrCAN/2(VehSpd) -> Gateway InfoCAN/2(VehSpd)
  connections:
  Two-Way Connection1/RConn1 -- Gateway_VehCAN/RConn1
  Gateway_InfoCAN/RConn1 -- Two-Way Connection/RConn1
  Gateway_PwtrCAN/RConn1 -- Two-Way Connection2/RConn1

== system CtrlStrct_CAN_Variant/CAN_Variant/VNT_Level_2_CAN/HEV_Ctrl ==
  note: HEV control
  note: HEV control
  note: CAN receive and transmit
  HEV_Ctrl_PwtrCAN Tx : Subsystem
  HEV_Ctrl_PwtrCAN_Rx : Subsystem
  Two-Way Connection : TwoWayConnection
  HevCtrl_PwtrCAN : PMIOPort  Side=Left
      settings: AttributesFormatString=<Side=%<Side>>
  tag scope: HEV_Ctrl_PwtrCAN_Rx=scoped
  wires:
  [HEV_Ctrl_PwtrCAN_Tx] -> HEV_Ctrl_PwtrCAN Tx/1(HEV_Ctrl_PwtrCAN_Tx_Apli)
  HEV_Ctrl_PwtrCAN Tx/1(HEV_Ctrl_PwtrCAN_Tx) -> Two-Way Connection/1
  Two-Way Connection/1 -> HEV_Ctrl_PwtrCAN_Rx/1(PwtrCAN)
  HEV_Ctrl_PwtrCAN_Rx/1(HEV_Ctrl_PwtrCAN_Rx) -> [HEV_Ctrl_PwtrCAN_Rx]
  connections:
  HevCtrl_PwtrCAN/RConn1 -- Two-Way Connection/RConn1

== system CtrlStrct_CAN_Variant/CAN_Variant/VNT_Level_2_CAN/HVAC_Ctrl ==
  note: HVAC control
  note: CAN receive and transmit
  note: HVAC Control
  HVAC_Ctrl_VehCAN Tx : Subsystem
  HVAC_Ctrl_VehCAN_Rx : Subsystem
  Two-Way Connection : TwoWayConnection
  HVAC_Ctrl_VehCAN : PMIOPort  Side=Right
      settings: AttributesFormatString=<Side=%<Side>>
  tag scope: HVAC_Ctrl_VehCAN_Rx=scoped
  wires:
  [HVAC_Ctrl_VehCAN_Tx] -> HVAC_Ctrl_VehCAN Tx/1(HVAC_Ctrl_VehCAN_Tx_Apli)
  HVAC_Ctrl_VehCAN Tx/1(HVAC_Ctrl_VehCAN_Tx) -> Two-Way Connection/1
  Two-Way Connection/1 -> HVAC_Ctrl_VehCAN_Rx/1(VehCAN)
  HVAC_Ctrl_VehCAN_Rx/1(HVAC_Ctrl_VehCAN_Rx) -> [HVAC_Ctrl_VehCAN_Rx]
  connections:
  HVAC_Ctrl_VehCAN/RConn1 -- Two-Way Connection/RConn1

== system CtrlStrct_CAN_Variant/CAN_Variant/VNT_Level_2_CAN/InfoCAN ==
  note: Infotainment CAN
  Bus Creator : BusCreator  Inputs=3
  Bus Selector : BusSelector  OutputSignals=NAVI_InfoCAN_Tx_0CFFB01C
  Bus Selector1 : BusSelector  OutputSignals=Gateway_InfoCAN_Tx_0CFFC485
  Bus Selector2 : BusSelector  OutputSignals=Radar_InfoCAN_Tx_0CFF0080
  CAN_Memory : Memory
  Two-Way Connection : TwoWayConnection
  Two-Way Connection1 : TwoWayConnection
  Two-Way Connection2 : TwoWayConnection
  NAVI_InfoCAN : PMIOPort  Side=Left
      settings: AttributesFormatString=<Side=%<Side>>
  Radar_InfoCAN : PMIOPort  Port=2  Side=Left
      settings: AttributesFormatString=<Side=%<Side>>
  Gateway_InfoCAN : PMIOPort  Port=3  Side=Right
      settings: AttributesFormatString=<Side=%<Side>>
  wires:
  Bus Creator/1 -> CAN_Memory/1  "InfoCAN"
  CAN_Memory/1 -> Two-Way Connection2/1, Two-Way Connection1/1, Two-Way Connection/1  "InfoCAN"
  Two-Way Connection/1 -> Bus Selector/1
  Two-Way Connection1/1 -> Bus Selector2/1
  Two-Way Connection2/1 -> Bus Selector1/1
  Bus Selector1/1 -> Bus Creator/1  "<Gateway_InfoCAN_Tx_0CFFC485>"
  Bus Selector/1 -> Bus Creator/2  "<NAVI_InfoCAN_Tx_0CFFB01C>"
  Bus Selector2/1 -> Bus Creator/3  "<Radar_InfoCAN_Tx_0CFF0080>"
  connections:
  Two-Way Connection/RConn1 -- NAVI_InfoCAN/RConn1
  Two-Way Connection1/RConn1 -- Radar_InfoCAN/RConn1
  Two-Way Connection2/RConn1 -- Gateway_InfoCAN/RConn1

== system CtrlStrct_CAN_Variant/CAN_Variant/VNT_Level_2_CAN/Motor_Ctrl ==
  note: Motor control
  note: Motor Control
  note: CAN receive and transmit
  MotorCtrl_PwtrCAN Tx : Subsystem
  MotorCtrl_PwtrCAN_Rx : Subsystem
  Two-Way Connection : TwoWayConnection
  MtrCtrl_PwtrCAN : PMIOPort  Side=Left
      settings: AttributesFormatString=<Side=%<Side>>
  tag scope: MotorCtrl_PwtrCAN_Rx=scoped
  wires:
  [MotorCtrl_PwtrCAN_Tx] -> MotorCtrl_PwtrCAN Tx/1(IMotorCtrl_PwtrCAN_Tx_Apli)
  MotorCtrl_PwtrCAN Tx/1(MotorCtrl_PwtrCAN_Tx_0CFF5083) -> Two-Way Connection/1
  Two-Way Connection/1 -> MotorCtrl_PwtrCAN_Rx/1(PwtrCAN)
  MotorCtrl_PwtrCAN_Rx/1(MotorCtrl_PwtrCAN_Rx) -> [MotorCtrl_PwtrCAN_Rx]
  connections:
  MtrCtrl_PwtrCAN/RConn1 -- Two-Way Connection/RConn1

== system CtrlStrct_CAN_Variant/CAN_Variant/VNT_Level_2_CAN/NAVI ==
  note: Navigation
  note: CAN receive and transmit
  note: Navigation
  NAVI_CAN_Rx : Subsystem
  NAVI_CAN_Tx : Subsystem
  Two-Way Connection : TwoWayConnection
  NAVI_InfoCAN : PMIOPort  Side=Right
      settings: AttributesFormatString=<Side=%<Side>>
  tag scope: NAVI_InfoCAN_Rx=scoped
  wires:
  NAVI_CAN_Rx/1(NAVI_InfoCAN_Rx) -> [NAVI_InfoCAN_Rx]  "NAVI_InfoCAN_Rx"
  [NAVI_InfoCAN_Tx] -> NAVI_CAN_Tx/1(NAVI_InfoCAN_Tx_Apli)
  NAVI_CAN_Tx/1(NAVI_InfoCAN_Tx) -> Two-Way Connection/1
  Two-Way Connection/1 -> NAVI_CAN_Rx/1(InfoCAN)
  connections:
  NAVI_InfoCAN/RConn1 -- Two-Way Connection/RConn1

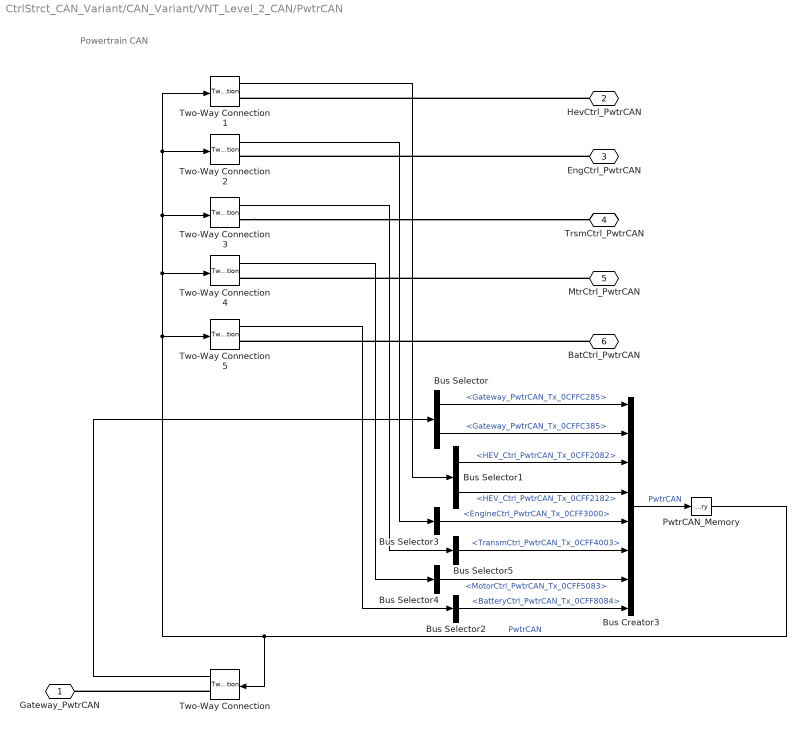
== system CtrlStrct_CAN_Variant/CAN_Variant/VNT_Level_2_CAN/PwtrCAN ==
  note: Powertrain CAN
  Bus Creator3 : BusCreator  Inputs=8
  Bus Selector : BusSelector  OutputSignals=Gateway_PwtrCAN_Tx_0CFFC285,Gateway_PwtrCAN_Tx_0CFFC385
  Bus Selector1 : BusSelector  OutputSignals=HEV_Ctrl_PwtrCAN_Tx_0CFF2082,HEV_Ctrl_PwtrCAN_Tx_0CFF2182
  Bus Selector2 : BusSelector  OutputSignals=BatteryCtrl_PwtrCAN_Tx_0CFF8084
  Bus Selector3 : BusSelector  OutputSignals=EngineCtrl_PwtrCAN_Tx_0CFF3000
  Bus Selector4 : BusSelector  OutputSignals=MotorCtrl_PwtrCAN_Tx_0CFF5083
  Bus Selector5 : BusSelector  OutputSignals=TransmCtrl_PwtrCAN_Tx_0CFF4003
  PwtrCAN_Memory : Memory
  Two-Way Connection{,1..5} (6 alike) : TwoWayConnection
  Gateway_PwtrCAN : PMIOPort  Side=Left
      settings: AttributesFormatString=<Side=%<Side>>
  HevCtrl_PwtrCAN : PMIOPort  Port=2  Side=Right
      settings: AttributesFormatString=<Side=%<Side>>
  EngCtrl_PwtrCAN : PMIOPort  Port=3  Side=Right
      settings: AttributesFormatString=<Side=%<Side>>
  TrsmCtrl_PwtrCAN : PMIOPort  Port=4  Side=Right
      settings: AttributesFormatString=<Side=%<Side>>
  MtrCtrl_PwtrCAN : PMIOPort  Port=5  Side=Right
      settings: AttributesFormatString=<Side=%<Side>>
  BatCtrl_PwtrCAN : PMIOPort  Port=6  Side=Right
      settings: AttributesFormatString=<Side=%<Side>>
  wires:
  Bus Creator3/1 -> PwtrCAN_Memory/1  "PwtrCAN"
  PwtrCAN_Memory/1 -> Two-Way Connection5/1, Two-Way Connection4/1, Two-Way Connection3/1, Two-Way Connection2/1, Two-Way Connection1/1, Two-Way Connection/1  "PwtrCAN"
  Two-Way Connection1/1 -> Bus Selector1/1
  Two-Way Connection/1 -> Bus Selector/1
  Two-Way Connection2/1 -> Bus Selector3/1
  Two-Way Connection5/1 -> Bus Selector2/1
  Two-Way Connection4/1 -> Bus Selector4/1
  Two-Way Connection3/1 -> Bus Selector5/1
  Bus Selector/1 -> Bus Creator3/1  "<Gateway_PwtrCAN_Tx_0CFFC285>"
  Bus Selector/2 -> Bus Creator3/2  "<Gateway_PwtrCAN_Tx_0CFFC385>"
  Bus Selector1/1 -> Bus Creator3/3  "<HEV_Ctrl_PwtrCAN_Tx_0CFF2082>"
  Bus Selector1/2 -> Bus Creator3/4  "<HEV_Ctrl_PwtrCAN_Tx_0CFF2182>"
  Bus Selector3/1 -> Bus Creator3/5  "<EngineCtrl_PwtrCAN_Tx_0CFF3000>"
  Bus Selector5/1 -> Bus Creator3/6  "<TransmCtrl_PwtrCAN_Tx_0CFF4003>"
  Bus Selector4/1 -> Bus Creator3/7  "<MotorCtrl_PwtrCAN_Tx_0CFF5083>"
  Bus Selector2/1 -> Bus Creator3/8  "<BatteryCtrl_PwtrCAN_Tx_0CFF8084>"
  connections:
  Two-Way Connection/RConn1 -- Gateway_PwtrCAN/RConn1
  HevCtrl_PwtrCAN/RConn1 -- Two-Way Connection1/RConn1
  EngCtrl_PwtrCAN/RConn1 -- Two-Way Connection2/RConn1
  Two-Way Connection3/RConn1 -- TrsmCtrl_PwtrCAN/RConn1
  MtrCtrl_PwtrCAN/RConn1 -- Two-Way Connection4/RConn1
  BatCtrl_PwtrCAN/RConn1 -- Two-Way Connection5/RConn1

== system CtrlStrct_CAN_Variant/CAN_Variant/VNT_Level_2_CAN/Radar ==
  note: Radar detection
  note: CAN receive and transmit
  note: Radar Detection
  Radar_CAN_Rx : Subsystem
  Radar_CAN_Tx : Subsystem
  Two-Way Connection : TwoWayConnection
  Radar_InfoCAN : PMIOPort  Side=Right
      settings: AttributesFormatString=<Side=%<Side>>
  tag scope: Radar_InfoCAN_Rx=scoped
  wires:
  [Radar_InfoCAN_Tx] -> Radar_CAN_Tx/1(Radar_InfoCAN_Tx_Apli)
  Radar_CAN_Tx/1(Radar_InfoCAN_Tx) -> Two-Way Connection/1
  Radar_CAN_Rx/1(Radar_InfoCAN_Rx) -> [Radar_InfoCAN_Rx]
  Two-Way Connection/1 -> Radar_CAN_Rx/1(InfoCAN)
  connections:
  Radar_InfoCAN/RConn1 -- Two-Way Connection/RConn1

== system CtrlStrct_CAN_Variant/CAN_Variant/VNT_Level_2_CAN/Steer_Ctrl ==
  note: Steering control
  note: CAN receive and transmit
  note: Steering Control
  SteerCtrl_VehCAN Tx : Subsystem
  SteerCtrl_VehCAN_Rx : Subsystem
  Two-Way Connection : TwoWayConnection
  StrCtrl_VehCAN : PMIOPort  Side=Right
      settings: AttributesFormatString=<Side=%<Side>>
  tag scope: SteerCtrl_VehCAN_Rx=scoped
  wires:
  [SteerCtrl_VehCAN_Tx] -> SteerCtrl_VehCAN Tx/1(SteerCtrl_VehCAN_Tx_Apli)
  SteerCtrl_VehCAN Tx/1(SteerCtrl_VehCAN_Tx) -> Two-Way Connection/1
  Two-Way Connection/1 -> SteerCtrl_VehCAN_Rx/1(VehCAN)
  SteerCtrl_VehCAN_Rx/1(SteerCtrl_VehCAN_Rx) -> [SteerCtrl_VehCAN_Rx]
  connections:
  StrCtrl_VehCAN/RConn1 -- Two-Way Connection/RConn1

== system CtrlStrct_CAN_Variant/CAN_Variant/VNT_Level_2_CAN/Transms_Ctrl ==
  note: Transmission control
  note: CAN receive and transmit
  note: Transmission Control
  TransmCtrl_PwtrCAN Tx : Subsystem
  TransmCtrl_PwtrCAN_Rx : Subsystem
  Two-Way Connection : TwoWayConnection
  TrsmCtrl_PwtrCAN : PMIOPort  Side=Left
      settings: AttributesFormatString=<Side=%<Side>>
  tag scope: TransmCtrl_PwtrCAN_Rx=scoped
  wires:
  [TransmCtrl_PwtrCAN_Tx] -> TransmCtrl_PwtrCAN Tx/1(TransmCtrl_PwtrCAN_Tx_Apli)
  TransmCtrl_PwtrCAN Tx/1(TransmCtrl_PwtrCAN_Tx) -> Two-Way Connection/1
  Two-Way Connection/1 -> TransmCtrl_PwtrCAN_Rx/1(PwtrCAN)
  TransmCtrl_PwtrCAN_Rx/1(TransmCtrl_PwtrCAN_Rx) -> [TransmCtrl_PwtrCAN_Rx]
  connections:
  TrsmCtrl_PwtrCAN/RConn1 -- Two-Way Connection/RConn1

== system CtrlStrct_CAN_Variant/CAN_Variant/VNT_Level_2_CAN/VM_Ctrl ==
  note: Vehicle motion control
  note: Vehicle Motion Control
  note: CAN receive and transmit
  Two-Way Connection : TwoWayConnection
  VM_Ctrl_VehCAN Tx : Subsystem
  VM_Ctrl_VehCAN_Rx : Subsystem
  VM_Ctrl_VehCAN : PMIOPort  Side=Right
      settings: AttributesFormatString=<Side=%<Side>>
  tag scope: VM_Ctrl_VehCAN_Rx=scoped
  wires:
  [VM_Ctrl_VehCAN_Tx] -> VM_Ctrl_VehCAN Tx/1(VM_Ctrl_VehCAN_Tx_Apli)
  VM_Ctrl_VehCAN Tx/1(VM_Ctrl_VehCAN_Tx) -> Two-Way Connection/1
  Two-Way Connection/1 -> VM_Ctrl_VehCAN_Rx/1(VehCAN)
  VM_Ctrl_VehCAN_Rx/1(VM_Ctrl_VehCAN_Rx) -> [VM_Ctrl_VehCAN_Rx]
  connections:
  VM_Ctrl_VehCAN/RConn1 -- Two-Way Connection/RConn1

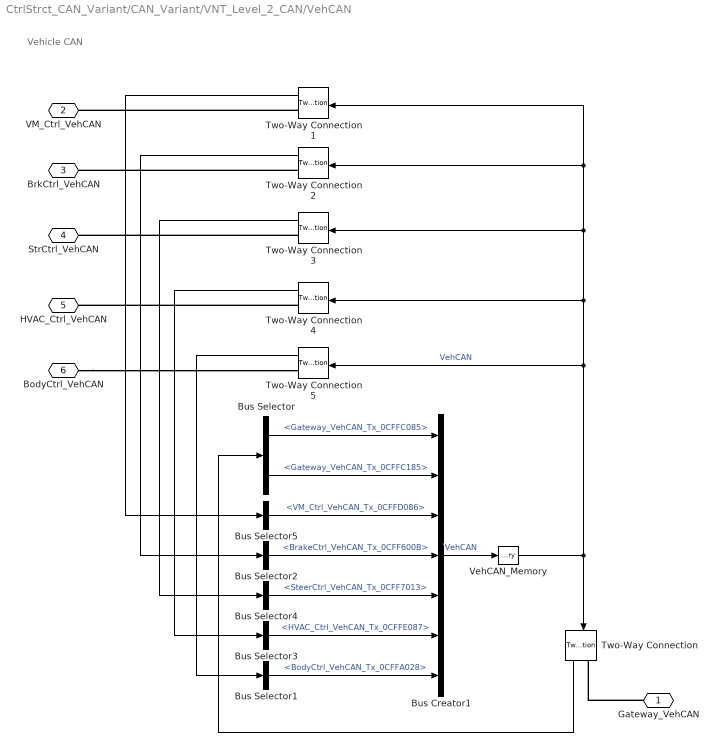
== system CtrlStrct_CAN_Variant/CAN_Variant/VNT_Level_2_CAN/VehCAN ==
  note: Vehicle CAN
  Bus Creator1 : BusCreator  Inputs=7
  Bus Selector : BusSelector  OutputSignals=Gateway_VehCAN_Tx_0CFFC085,Gateway_VehCAN_Tx_0CFFC185
  Bus Selector1 : BusSelector  OutputSignals=BodyCtrl_VehCAN_Tx_0CFFA028
  Bus Selector2 : BusSelector  OutputSignals=BrakeCtrl_VehCAN_Tx_0CFF600B
  Bus Selector3 : BusSelector  OutputSignals=HVAC_Ctrl_VehCAN_Tx_0CFFE087
  Bus Selector4 : BusSelector  OutputSignals=SteerCtrl_VehCAN_Tx_0CFF7013
  Bus Selector5 : BusSelector  OutputSignals=VM_Ctrl_VehCAN_Tx_0CFFD086
  Two-Way Connection{,1..5} (6 alike) : TwoWayConnection
  VehCAN_Memory : Memory
  Gateway_VehCAN : PMIOPort  Side=Right
      settings: AttributesFormatString=<Side=%<Side>>
  VM_Ctrl_VehCAN : PMIOPort  Port=2  Side=Left
      settings: AttributesFormatString=<Side=%<Side>>
  BrkCtrl_VehCAN : PMIOPort  Port=3  Side=Left
      settings: AttributesFormatString=<Side=%<Side>>
  StrCtrl_VehCAN : PMIOPort  Port=4  Side=Left
      settings: AttributesFormatString=<Side=%<Side>>
  HVAC_Ctrl_VehCAN : PMIOPort  Port=5  Side=Left
      settings: AttributesFormatString=<Side=%<Side>>
  BodyCtrl_VehCAN : PMIOPort  Port=6  Side=Left
      settings: AttributesFormatString=<Side=%<Side>>
  wires:
  Bus Creator1/1 -> VehCAN_Memory/1  "VehCAN"
  Two-Way Connection3/1 -> Bus Selector4/1
  Two-Way Connection1/1 -> Bus Selector5/1
  Two-Way Connection5/1 -> Bus Selector1/1
  VehCAN_Memory/1 -> Two-Way Connection4/1, Two-Way Connection3/1, Two-Way Connection2/1, Two-Way Connection1/1, Two-Way Connection5/1, Two-Way Connection/1  "VehCAN"
  Two-Way Connection2/1 -> Bus Selector2/1
  Two-Way Connection/1 -> Bus Selector/1
  Two-Way Connection4/1 -> Bus Selector3/1
  Bus Selector/1 -> Bus Creator1/1  "<Gateway_VehCAN_Tx_0CFFC085>"
  Bus Selector/2 -> Bus Creator1/2  "<Gateway_VehCAN_Tx_0CFFC185>"
  Bus Selector5/1 -> Bus Creator1/3  "<VM_Ctrl_VehCAN_Tx_0CFFD086>"
  Bus Selector2/1 -> Bus Creator1/4  "<BrakeCtrl_VehCAN_Tx_0CFF600B>"
  Bus Selector4/1 -> Bus Creator1/5  "<SteerCtrl_VehCAN_Tx_0CFF7013>"
  Bus Selector3/1 -> Bus Creator1/6  "<HVAC_Ctrl_VehCAN_Tx_0CFFE087>"
  Bus Selector1/1 -> Bus Creator1/7  "<BodyCtrl_VehCAN_Tx_0CFFA028>"
  connections:
  Gateway_VehCAN/RConn1 -- Two-Way Connection/RConn1
  Two-Way Connection1/RConn1 -- VM_Ctrl_VehCAN/RConn1
  Two-Way Connection2/RConn1 -- BrkCtrl_VehCAN/RConn1
  Two-Way Connection3/RConn1 -- StrCtrl_VehCAN/RConn1
  Two-Way Connection4/RConn1 -- HVAC_Ctrl_VehCAN/RConn1
  BodyCtrl_VehCAN/RConn1 -- Two-Way Connection5/RConn1

== system CtrlStrct_CAN_Variant/Powertrain/Engine_Control/Engine_Control ==
  "DrvDem " : Inport
  "Eng_Sns " : Inport  Port=2
  EngineCtrl_PwtrCAN_Rx : Inport  Port=3
  "Info_in " : Inport  Port=4
  EngineCtrl_V1.slx : ModelReference  ModelNameDialog=EngineCtrl_V1_1.slx  SimulationMode=Normal  VariantControl=VarObj_EngEcu_Simple  ModelReferenceVersion=1.0.25
  EngineCtrl_V2.slx : ModelReference  ModelNameDialog=EngineCtrl_V2.slx  SimulationMode=Normal  VariantControl=VarObj_EngEcu_Medium  ModelReferenceVersion=1.0.8
  " EngineCtrl" : Outport
  " EngineCtrl_PwtrCAN_Tx" : Outport  Port=2
  " EngineCtrl_Info" : Outport  Port=3
